simulink model "OffboardAPI"  (R2021b)
settings: Solver=ode4  StartTime=0.0  StopTime=inf  FixedStep=0.01  RelTol=1e-3
PreLoadFcn:
  | filepath  = fileparts(get_param(bdroot, 'FileName'))
  | cd(filepath);
undefined symbols (not defined in the file): Busy, Earth, Wait, WGS84
libraries: etargetslib x10, slrealtimeiplib x2, dspnetwork x2, slrealtimeutilitieslib x1, aerolibanimutils x1, aerolibtransform2 x1
settings Model: Creator=dream  LastModifiedBy=Lenovo
settings SolverCC: AlgebraicLoopSolver=TrustRegion
settings DataIOCC: ReturnWorkspaceOutputs=off
settings DebuggingCC: SFMachineParentedDataDiag=warning  ArithmeticOperatorsInVariantConditions=warning
settings SFSimCC: SimUseLocalCustomCode=off  CustomCodeUndefinedFunction=UseInterfaceOnly
settings RTWCC: RTWUseLocalCustomCode=off

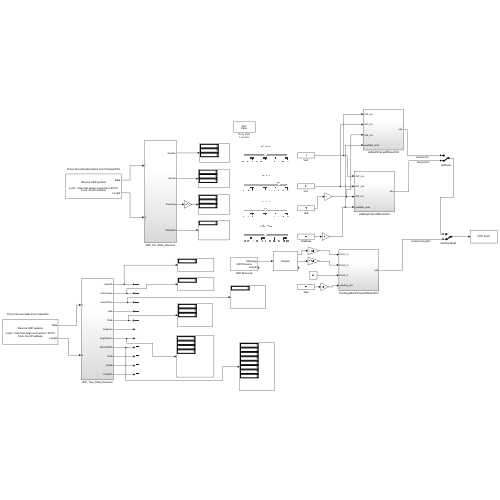
[thumbnail: Simulink's stored preview of the top-level diagram]
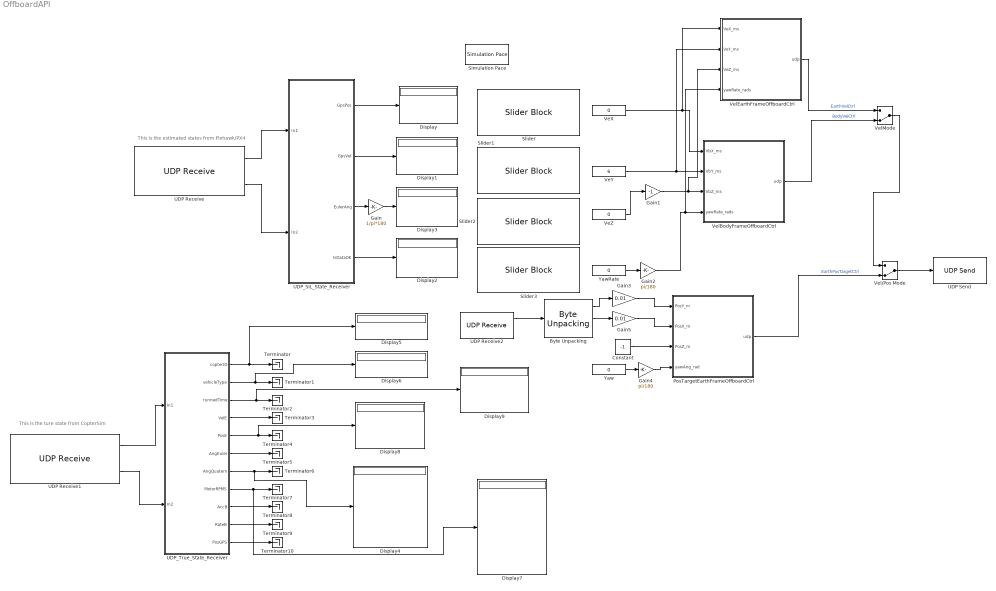
== system OffboardAPI ==
  note: This is the estimated states from Pixhawk/PX4
  note: This is the ture state from CopterSim
  Byte Unpacking : slrealtimeutilitieslib/Byte Unpacking  MaskUnpackedDataTypes={'double','double','double'}  MaskUnpackedDataSizes={[1],[1],[1]}  MaskAlignment=1
      settings: SourceProductBaseCode=XP
  Constant : Constant  Value=-1
  Display{,1..9} (10 alike) : Display
  Gain : Gain  Gain=1/pi*180
  Gain1 : Gain  Gain=-1
  Gain2 : Gain  Gain=pi/180
  Gain3 : Gain  Gain=0.01
  Gain4 : Gain  Gain=pi/180
  Gain5 : Gain  Gain=0.01
  PosTargetEarthFrameOffboardCtrl : Subsystem
  Simulation Pace : aerolibanimutils/Simulation Pace  SimulationPace=1  SleepMode=Busy-Wait  OutputPaceError=off  SampleTime=-1
  Slider : SliderBlock  ScaleMin=-10  ScaleMax=10
  Slider1 : SliderBlock  ScaleMin=-10  ScaleMax=10
  Slider2 : SliderBlock  ScaleMin=-10  ScaleMax=10
  Slider3 : SliderBlock  ScaleMin=-180  ScaleMax=180
  Terminator{,1..10} (11 alike) : Terminator
  UDP Receive : slrealtimeiplib/UDP Receive  useHostTargetConn=on  ipAddress=10.10.10.15  localPort=20101  rcvWidth=125  rcvFmAny=on  fmAddress=0.0.0.0  sampleTime=-1
      settings: SourceProductBaseCode=XP
  UDP Receive1 : slrealtimeiplib/UDP Receive  useHostTargetConn=on  ipAddress=10.10.10.15  localPort=30101  rcvWidth=250  rcvFmAny=on  fmAddress=0.0.0.0  sampleTime=-1
      settings: SourceProductBaseCode=XP
  UDP Receive2 : dspnetwork/UDP Receive  localURL='0.0.0.0'  localPort=1230  remoteURL='127.0.0.1'  remotePort=-1  recvBufferSize=24  dims=3  signalDatatype=double  isComplex=off  isVarSize=off  showBlockingTime=off  blockingTime=0  sampletime=-1  blockPlatform=[]
  UDP Send : dspnetwork/UDP Send  remoteURL='127.0.0.1'  remotePort=20100  localURL='0.0.0.0'  localPortSource=Automatically determine  localPort=-1  sendBufferSize=8192  sampletime=-1  blockPlatform=[]  separateLengthPort=0
  UDP_SIL_State_Receiver : Subsystem
  UDP_True_State_Receiver : Subsystem
  VeX : Constant  Value=0
  VeY : Constant  Value=6
  VeZ : Constant  Value=0
  Vel/Pos Mode : ManualSwitch  CurrentSetting=0
  VelBodyFrameOffboardCtrl : Subsystem
  VelEarthFrameOffboardCtrl : Subsystem
  VelMode : ManualSwitch  CurrentSetting=0
  Yaw : Constant  Value=0
  YawRate : Constant  Value=0
  wires:
  UDP Receive/1 -> UDP_SIL_State_Receiver/1(In1)
  UDP Receive/2 -> UDP_SIL_State_Receiver/2(In2)
  UDP_SIL_State_Receiver/1(GpsPos) -> Display/1
  UDP_SIL_State_Receiver/2(GpsVel) -> Display1/1
  UDP_SIL_State_Receiver/3(EulerAng) -> Gain/1
  VeX/1 -> VelEarthFrameOffboardCtrl/1(VeX_ms), VelBodyFrameOffboardCtrl/1(VbX_ms)
  VeY/1 -> VelEarthFrameOffboardCtrl/2(VeY_ms), VelBodyFrameOffboardCtrl/2(VbY_ms)
  VeZ/1 -> Gain1/1
  YawRate/1 -> Gain2/1
  VelBodyFrameOffboardCtrl/1(udp) -> VelMode/2  "BodyVelCtrl"
  Gain/1 -> Display3/1
  Gain1/1 -> VelEarthFrameOffboardCtrl/3(VeZ_ms), VelBodyFrameOffboardCtrl/3(VbZ_ms)
  UDP_SIL_State_Receiver/4(IsDataOK) -> Display2/1
  Gain2/1 -> VelEarthFrameOffboardCtrl/4(yawRate_rads), VelBodyFrameOffboardCtrl/4(yawRate_rads)
  Yaw/1 -> Gain4/1
  PosTargetEarthFrameOffboardCtrl/1(udp) -> Vel/Pos Mode/2  "EarthPosTargetCtrl"
  Vel/Pos Mode/1 -> UDP Send/1
  Gain4/1 -> PosTargetEarthFrameOffboardCtrl/4(yawAng_rad)
  VelEarthFrameOffboardCtrl/1(udp) -> VelMode/1  "EarthVelCtrl"
  VelMode/1 -> Vel/Pos Mode/1
  UDP_True_State_Receiver/2(vehicleType) -> Display6/1, Terminator1/1
  UDP Receive1/2 -> UDP_True_State_Receiver/2(In2)
  UDP_True_State_Receiver/11(PosGPS) -> Terminator10/1
  UDP_True_State_Receiver/10(RateB) -> Terminator9/1
  UDP_True_State_Receiver/8(MotorRPMS) -> Display7/1, Terminator7/1
  UDP_True_State_Receiver/9(AccB) -> Terminator8/1
  UDP_True_State_Receiver/1(copterID) -> Display5/1, Terminator/1
  UDP_True_State_Receiver/7(AngQuatern) -> Display4/1, Terminator6/1
  UDP_True_State_Receiver/3(runnedTime) -> Display9/1, Terminator2/1
  UDP_True_State_Receiver/5(PosE) -> Display8/1, Terminator4/1
  UDP_True_State_Receiver/6(AngEuler) -> Terminator5/1
  UDP_True_State_Receiver/4(VelE) -> Terminator3/1
  UDP Receive1/1 -> UDP_True_State_Receiver/1(In1)
  Byte Unpacking/1 -> Gain3/1
  Byte Unpacking/2 -> Gain5/1
  UDP Receive2/1 -> Byte Unpacking/1
  Gain3/1 -> PosTargetEarthFrameOffboardCtrl/1(PosY_m)
  Gain5/1 -> PosTargetEarthFrameOffboardCtrl/2(PosX_m)
  Constant/1 -> PosTargetEarthFrameOffboardCtrl/3(PosZ_m)

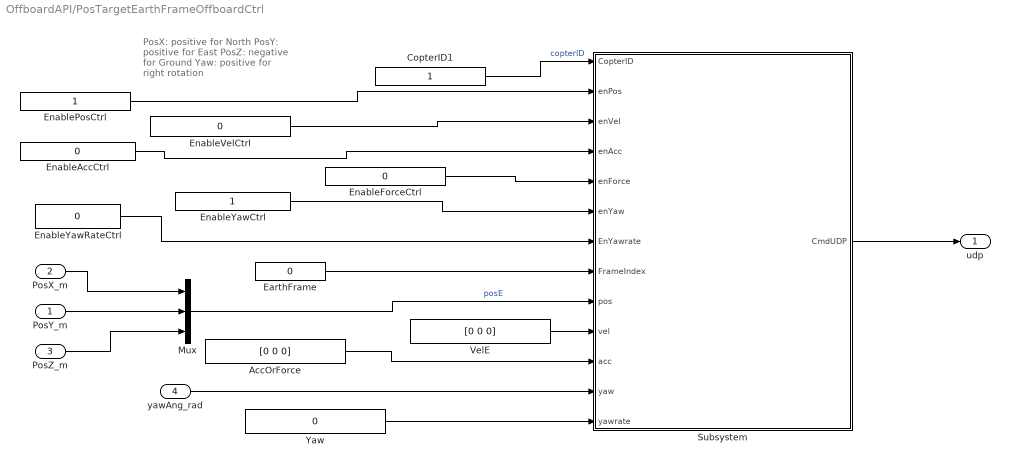
== system OffboardAPI/PosTargetEarthFrameOffboardCtrl ==
  note: PosX: positive for North
      | PosY: positive for East
      | PosZ: negative for Ground
      | Yaw: positive for right rotation
  PosY_m : Inport
  PosX_m : Inport  Port=2
  PosZ_m : Inport  Port=3
  yawAng_rad : Inport  Port=4  PortDimensions=1
  AccOrForce : Constant  Value=[0 0 0]
  CopterID1 : Constant
  EarthFrame : Constant  Value=0
  EnableAccCtrl : Constant  Value=0
  EnableForceCtrl : Constant  Value=0
  EnablePosCtrl : Constant
  EnableVelCtrl : Constant  Value=0
  EnableYawCtrl : Constant
  EnableYawRateCtrl : Constant  Value=0
  Mux : Mux  Inputs=3
  Subsystem : Subsystem
  VelE : Constant  Value=[0 0 0]
  Yaw : Constant  Value=0
  udp : Outport  VectorParamsAs1DForOutWhenUnconnected=off
  wires:
  Subsystem/1(CmdUDP) -> udp/1
  Yaw/1 -> Subsystem/13(yawrate)
  EnableYawRateCtrl/1 -> Subsystem/7(EnYawrate)
  EnableYawCtrl/1 -> Subsystem/6(enYaw)
  EnableAccCtrl/1 -> Subsystem/4(enAcc)
  Mux/1 -> Subsystem/9(pos)  "posE"
  EarthFrame/1 -> Subsystem/8(FrameIndex)
  yawAng_rad/1 -> Subsystem/12(yaw)
  AccOrForce/1 -> Subsystem/11(acc)
  EnableVelCtrl/1 -> Subsystem/3(enVel)
  EnableForceCtrl/1 -> Subsystem/5(enForce)
  CopterID1/1 -> Subsystem/1(CopterID)  "copterID"
  EnablePosCtrl/1 -> Subsystem/2(enPos)
  VelE/1 -> Subsystem/10(vel)
  PosY_m/1 -> Mux/2
  PosX_m/1 -> Mux/1
  PosZ_m/1 -> Mux/3

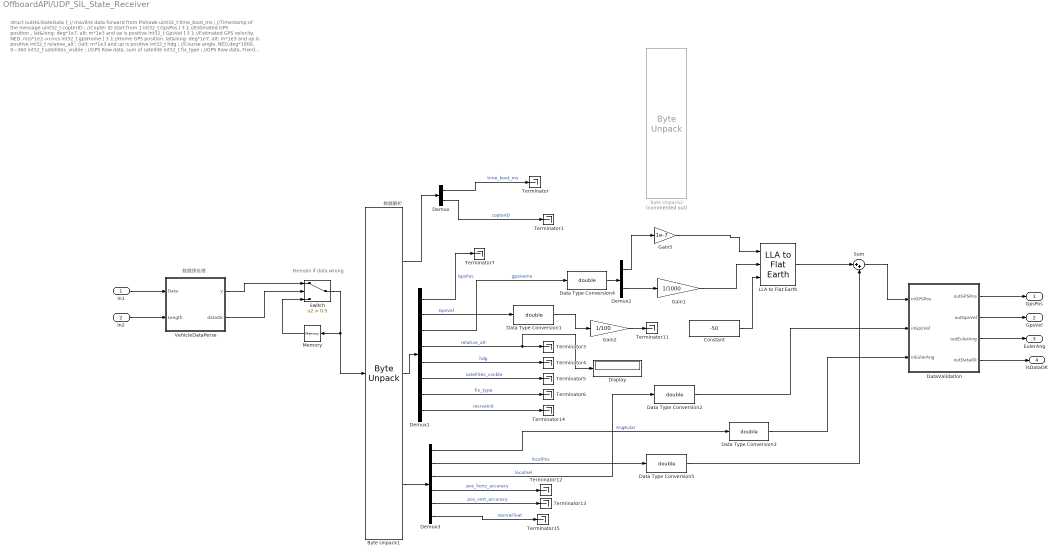
== system OffboardAPI/UDP_SIL_State_Receiver ==
  note: 数据解析
  note: 数据预处理
  note: Remain if data wrong
  note: struct outHILStateData { // mavlink data forward from Pixhawk
      | uint32_t time_boot_ms ; //Timestamp of the message
      | uint32_t copterID ; //Copter ID start from 1
      | int32_t GpsPos [ 3 ]; //Estimated GPS position，lat&long: deg*1e7, alt: m*1e3 and up is positive
      | int32_t GpsVel [ 3 ]; //Estimated GPS velocity, NED, m/s*1e2->cm/s
      | int32_t gpsHome [ 3 ]; //Home GPS position, lat&long: deg*1e7, alt: m*1e3 and up is positive
      | int32_t relative_alt ; //alt: m*1e3 and up is positive
      | int32_t hdg ; //Course angle, NED,deg*1000, 0~360
      | int32_t satellites_visible ; //GPS Raw data, sum of satellite
      | int32_t fix_type ; //GPS Raw data, Fixed type, 3 for fixed (good precision)
      | int32_t resrveInit ; //Int, reserve for the future use
      | float AngEular [ 3 ]; //Estimated Euler angle, unit: rad/s
      | float localPos [ 3 ]; //Estimated locoal position, NED, unit: m
      | float localVel [ 3 ]; //Estimated locoal velocity, NED, unit: m/s
      | float pos_horiz_accuracy ; //GPS horizontal accuracy, unit: m
      | float pos_vert_accuracy ; //GPS vertical accuracy, unit: m
      | float resrveFloat ; //float,reserve for the future use
      | }
  In1 : Inport
  In2 : Inport  Port=2
  Byte Unpack1 : etargetslib/Byte Unpack  dimensions={2,14,12}  datatypes={'uint32','int32','single'}  byteAlign=8
  Byte Unpack2 : etargetslib/Byte Unpack  Commented=on  dimensions={1,1,1,3,3,3,4,8,3,3,3}  datatypes={'int32','int32','double','single','single','single','single','single','single','single','double'}  byteAlign=1
  Constant : Constant  Value=-50
  Data Type Conversion{1..5} (5 alike) : DataTypeConversion  OutDataTypeStr=double
  DataValidation : MATLAB Function  TreatAsAtomicUnit=on
  Demux : Demux  Outputs=2
  Demux1 : Demux  Outputs=[3,3,3,1,1,1,1,1]
  Demux2 : Demux  Outputs=[2,1]
  Demux3 : Demux  Outputs=[3,3,3,1,1,1]
  Display : Display
  Gain1 : Gain  Gain=1/1000
  Gain2 : Gain  Gain=1/100
  Gain5 : Gain  Gain=1e-7
  LLA to Flat Earth : aerolibtransform2/LLA to Flat Earth  units=Metric (MKS)  ptype=Earth (WGS84)  F=1/298.257223563  R=6378137  refPosPort=off  LL0=[40.1540302 116.259368300000]  psi=0
      settings: SourceProductBaseCode=AE
  Memory : Memory  InitialCondition=uint8(zeros(112,1))
  Sum : Sum  Inputs=|++
  Switch : Switch  Criteria=u2 > Threshold  Threshold=0.5
  Terminator{,1,3..7,11..15} (12 alike) : Terminator
  VehicleDataPerse : MATLAB Function  TreatAsAtomicUnit=on
  GpsPos : Outport  VectorParamsAs1DForOutWhenUnconnected=off
  GpsVel : Outport  Port=2  VectorParamsAs1DForOutWhenUnconnected=off
  EulerAng : Outport  Port=3  VectorParamsAs1DForOutWhenUnconnected=off
  IsDataOK : Outport  Port=4  VectorParamsAs1DForOutWhenUnconnected=off
  wires:
  VehicleDataPerse/2(dataOk) -> Switch/2
  In2/1 -> VehicleDataPerse/2(Length)
  In1/1 -> VehicleDataPerse/1(Data)
  VehicleDataPerse/1(y) -> Switch/1
  Switch/1 -> Memory/1, Byte Unpack1/1
  Memory/1 -> Switch/3
  Byte Unpack1/1 -> Demux/1
  Demux/1 -> Terminator/1  "time_boot_ms"
  Demux/2 -> Terminator1/1  "copterID"
  Byte Unpack1/2 -> Demux1/1
  Demux1/2 -> Data Type Conversion1/1  "GpsVel"
  Demux2/1 -> Gain5/1
  Demux2/2 -> Gain1/1
  Gain1/1 -> LLA to Flat Earth/2
  Demux1/1 -> Terminator7/1  "GpsPos"
  LLA to Flat Earth/1 -> Sum/1
  Data Type Conversion1/1 -> Gain2/1
  Data Type Conversion3/1 -> DataValidation/3(inEulerAng)
  Gain5/1 -> LLA to Flat Earth/1
  Data Type Conversion4/1 -> Demux2/1
  Byte Unpack1/3 -> Demux3/1
  Demux1/3 -> Data Type Conversion4/1  "gpsHome"
  Demux1/4 -> Display/1, Terminator3/1  "relative_alt"
  Demux1/5 -> Terminator4/1  "hdg"
  Demux1/6 -> Terminator5/1  "satellites_visible"
  Demux1/7 -> Terminator6/1  "fix_type"
  Demux3/1 -> Data Type Conversion3/1  "AngEular"
  Demux3/2 -> Data Type Conversion5/1  "localPos"
  Demux3/3 -> Data Type Conversion2/1  "localVel"
  Demux3/4 -> Terminator12/1  "pos_horiz_accuracy"
  Demux3/5 -> Terminator13/1  "pos_vert_accuracy"
  Demux1/8 -> Terminator14/1  "resrveInit"
  Demux3/6 -> Terminator15/1  "resrveFloat"
  Constant/1 -> LLA to Flat Earth/3
  DataValidation/1(outGPSPos) -> GpsPos/1
  DataValidation/2(outGpsVel) -> GpsVel/1
  DataValidation/3(outEulerAng) -> EulerAng/1
  DataValidation/4(outDataOk) -> IsDataOK/1
  Data Type Conversion2/1 -> DataValidation/2(inGpsVel)
  Gain2/1 -> Terminator11/1
  Data Type Conversion5/1 -> Sum/2
  Sum/1 -> DataValidation/1(inGPSPos)

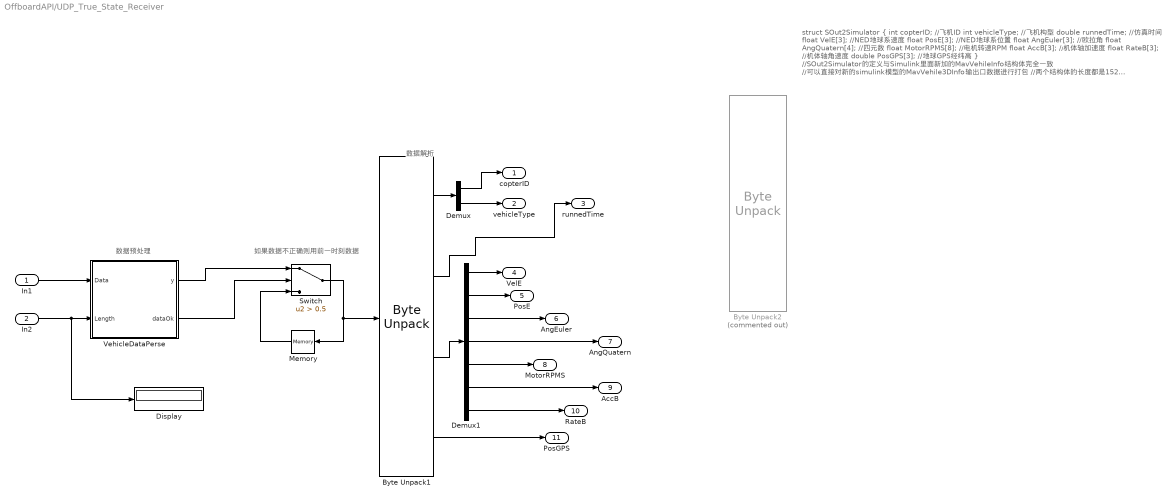
== system OffboardAPI/UDP_True_State_Receiver ==
  note: 数据解析
  note: 数据预处理
  note: 如果数据不正确则用前一时刻数据
  note: struct SOut2Simulator
      | {
      | int copterID; //飞机ID
      | int vehicleType; //飞机构型
      | double runnedTime; //仿真时间
      | float VelE[3]; //NED地球系速度
      | float PosE[3]; //NED地球系位置
      | float AngEuler[3]; //欧拉角
      | float AngQuatern[4]; //四元数
      | float MotorRPMS[8]; //电机转速RPM
      | float AccB[3]; //机体轴加速度
      | float RateB[3]; //机体轴角速度
      | double PosGPS[3]; //地球GPS经纬高
      | }
      |
      | //SOut2Simulator的定义与Simulink里面新加的MavVehileInfo结构体完全一致
      | //可以直接对新的simulink模型的MavVehile3DInfo输出口数据进行打包
      | //两个结构体的长度都是152
      | sizeof(SOut2Simulator) = sizeof(MavVehileInfo) = 152
      |
      | 打包封装的结构体为
      | typedef struct _netDataShort
      | {
      | TargetType tg; //这里目前随便填，写1即可 uint32
      | int len; //这个长度为传输结构体长度，目前是152
      | char payload[192]; //这里面前152位存放了SOut2Simulator结构体数据，后面的40位保留
      | }netDataShort;
      |
      | //UDP包的总长度为200
      | sizeof(netDataShort) = 200
      |
      | //发送的UDP端口号为：20010
  In1 : Inport
  In2 : Inport  Port=2
  Byte Unpack1 : etargetslib/Byte Unpack  dimensions={2,1,27,3}  datatypes={'int32','double','single','double'}  byteAlign=8
  Byte Unpack2 : etargetslib/Byte Unpack  Commented=on  dimensions={1,1,1,3,3,3,4,8,3,3,3}  datatypes={'int32','int32','double','single','single','single','single','single','single','single','double'}  byteAlign=1
  Demux : Demux  Outputs=2
  Demux1 : Demux  Outputs=[3,3,3,4,8,3,3]
  Display : Display
  Memory : Memory  InitialCondition=uint8(zeros(152,1))
  Switch : Switch  Criteria=u2 > Threshold  Threshold=0.5
  VehicleDataPerse : MATLAB Function  TreatAsAtomicUnit=on
  copterID : Outport  VectorParamsAs1DForOutWhenUnconnected=off
  vehicleType : Outport  Port=2  VectorParamsAs1DForOutWhenUnconnected=off
  runnedTime : Outport  Port=3  VectorParamsAs1DForOutWhenUnconnected=off
  VelE : Outport  Port=4  VectorParamsAs1DForOutWhenUnconnected=off
  PosE : Outport  Port=5  VectorParamsAs1DForOutWhenUnconnected=off
  AngEuler : Outport  Port=6  VectorParamsAs1DForOutWhenUnconnected=off
  AngQuatern : Outport  Port=7  VectorParamsAs1DForOutWhenUnconnected=off
  MotorRPMS : Outport  Port=8  VectorParamsAs1DForOutWhenUnconnected=off
  AccB : Outport  Port=9  VectorParamsAs1DForOutWhenUnconnected=off
  RateB : Outport  Port=10  VectorParamsAs1DForOutWhenUnconnected=off
  PosGPS : Outport  Port=11  VectorParamsAs1DForOutWhenUnconnected=off
  wires:
  VehicleDataPerse/2(dataOk) -> Switch/2
  In2/1 -> Display/1, VehicleDataPerse/2(Length)
  In1/1 -> VehicleDataPerse/1(Data)
  VehicleDataPerse/1(y) -> Switch/1
  Switch/1 -> Memory/1, Byte Unpack1/1
  Memory/1 -> Switch/3
  Byte Unpack1/1 -> Demux/1
  Demux/1 -> copterID/1
  Demux/2 -> vehicleType/1
  Byte Unpack1/2 -> runnedTime/1
  Byte Unpack1/3 -> Demux1/1
  Demux1/1 -> VelE/1
  Demux1/2 -> PosE/1
  Demux1/3 -> AngEuler/1
  Demux1/4 -> AngQuatern/1
  Demux1/5 -> MotorRPMS/1
  Demux1/6 -> AccB/1
  Demux1/7 -> RateB/1
  Byte Unpack1/4 -> PosGPS/1

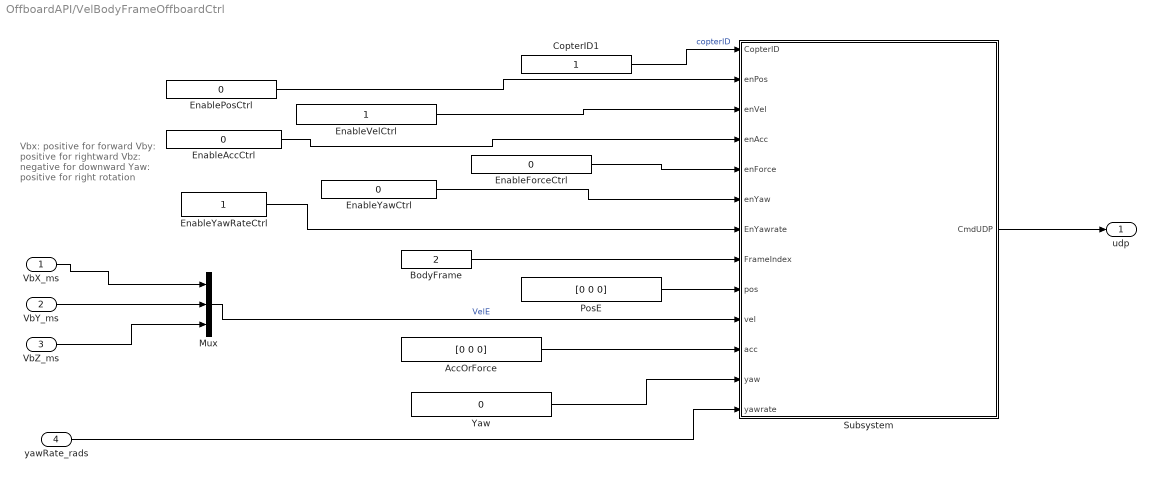
== system OffboardAPI/VelBodyFrameOffboardCtrl ==
  note: Vbx: positive for forward
      | Vby: positive for rightward
      | Vbz: negative for downward
      | Yaw: positive for right rotation
  VbX_ms : Inport
  VbY_ms : Inport  Port=2
  VbZ_ms : Inport  Port=3
  yawRate_rads : Inport  Port=4  PortDimensions=1
  AccOrForce : Constant  Value=[0 0 0]
  BodyFrame : Constant  Value=2
  CopterID1 : Constant
  EnableAccCtrl : Constant  Value=0
  EnableForceCtrl : Constant  Value=0
  EnablePosCtrl : Constant  Value=0
  EnableVelCtrl : Constant
  EnableYawCtrl : Constant  Value=0
  EnableYawRateCtrl : Constant
  Mux : Mux  Inputs=3
  PosE : Constant  Value=[0 0 0]
  Subsystem : Subsystem
  Yaw : Constant  Value=0
  udp : Outport  VectorParamsAs1DForOutWhenUnconnected=off
  wires:
  Subsystem/1(CmdUDP) -> udp/1
  Yaw/1 -> Subsystem/12(yaw)
  EnableYawRateCtrl/1 -> Subsystem/7(EnYawrate)
  EnableYawCtrl/1 -> Subsystem/6(enYaw)
  EnableAccCtrl/1 -> Subsystem/4(enAcc)
  Mux/1 -> Subsystem/10(vel)  "VelE"
  BodyFrame/1 -> Subsystem/8(FrameIndex)
  yawRate_rads/1 -> Subsystem/13(yawrate)
  AccOrForce/1 -> Subsystem/11(acc)
  EnableVelCtrl/1 -> Subsystem/3(enVel)
  EnableForceCtrl/1 -> Subsystem/5(enForce)
  CopterID1/1 -> Subsystem/1(CopterID)  "copterID"
  EnablePosCtrl/1 -> Subsystem/2(enPos)
  PosE/1 -> Subsystem/9(pos)
  VbY_ms/1 -> Mux/2
  VbX_ms/1 -> Mux/1
  VbZ_ms/1 -> Mux/3

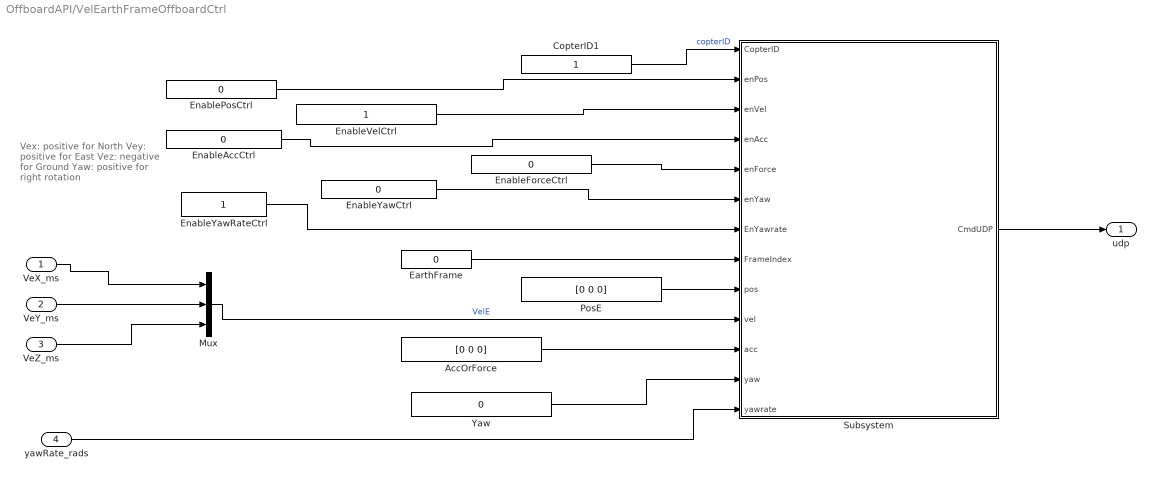
== system OffboardAPI/VelEarthFrameOffboardCtrl ==
  note: Vex: positive for North
      | Vey: positive for East
      | Vez: negative for Ground
      | Yaw: positive for right rotation
  VeX_ms : Inport
  VeY_ms : Inport  Port=2
  VeZ_ms : Inport  Port=3
  yawRate_rads : Inport  Port=4  PortDimensions=1
  AccOrForce : Constant  Value=[0 0 0]
  CopterID1 : Constant
  EarthFrame : Constant  Value=0
  EnableAccCtrl : Constant  Value=0
  EnableForceCtrl : Constant  Value=0
  EnablePosCtrl : Constant  Value=0
  EnableVelCtrl : Constant
  EnableYawCtrl : Constant  Value=0
  EnableYawRateCtrl : Constant
  Mux : Mux  Inputs=3
  PosE : Constant  Value=[0 0 0]
  Subsystem : Subsystem
  Yaw : Constant  Value=0
  udp : Outport  VectorParamsAs1DForOutWhenUnconnected=off
  wires:
  Subsystem/1(CmdUDP) -> udp/1
  Yaw/1 -> Subsystem/12(yaw)
  EnableYawRateCtrl/1 -> Subsystem/7(EnYawrate)
  EnableYawCtrl/1 -> Subsystem/6(enYaw)
  EnableAccCtrl/1 -> Subsystem/4(enAcc)
  Mux/1 -> Subsystem/10(vel)  "VelE"
  EarthFrame/1 -> Subsystem/8(FrameIndex)
  yawRate_rads/1 -> Subsystem/13(yawrate)
  AccOrForce/1 -> Subsystem/11(acc)
  EnableVelCtrl/1 -> Subsystem/3(enVel)
  EnableForceCtrl/1 -> Subsystem/5(enForce)
  CopterID1/1 -> Subsystem/1(CopterID)  "copterID"
  EnablePosCtrl/1 -> Subsystem/2(enPos)
  PosE/1 -> Subsystem/9(pos)
  VeY_ms/1 -> Mux/2
  VeX_ms/1 -> Mux/1
  VeZ_ms/1 -> Mux/3

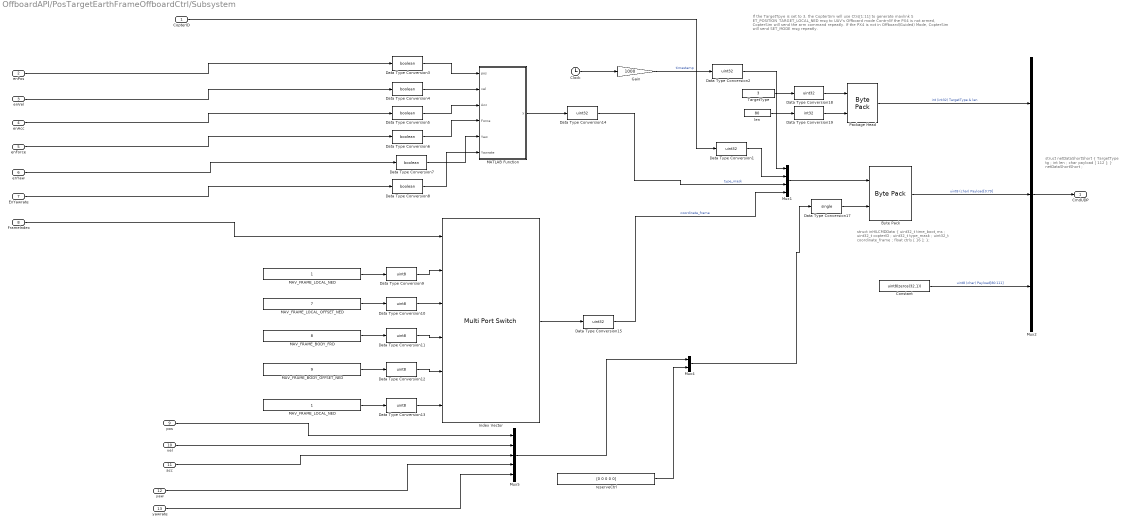
== system OffboardAPI/PosTargetEarthFrameOffboardCtrl/Subsystem ==
  note: struct netDataShortShort {
      | TargetType tg ;
      | int len ;
      | char payload [ 112 ];
      | } netDataShortShort ;
  note: struct inHILCMDData {
      | uint32_t time_boot_ms ;
      | uint32_t copterID ;
      | uint32_t type_mask ;
      | uint32_t coordinate_frame ;
      | float ctrls [ 16 ];
      | };
  note: If the TargetTpye is set to 3, the CopterSim will use Ctrs[1:11] to generate mavlink S ET_POSITION_TARGET_LOCAL_NED msg to UAV's Offboard mode Control，
      | If the PX4 is not armed, CopterSim will send the arm command repeatly. If the PX4 is not in Offboard(Guided) Mode, CopterSim will send SET_MODE msg repeatly.
  CopterID : Inport
  enPos : Inport  Port=2
  enVel : Inport  Port=3
  enAcc : Inport  Port=4
  enForce : Inport  Port=5
  enYaw : Inport  Port=6
  EnYawrate : Inport  Port=7
  FrameIndex : Inport  Port=8
  pos : Inport  Port=9  PortDimensions=3
  vel : Inport  Port=10  PortDimensions=3
  acc : Inport  Port=11  PortDimensions=3
  yaw : Inport  Port=12  PortDimensions=1
  yawrate : Inport  Port=13  PortDimensions=1
  Byte Pack : etargetslib/Byte Pack  datatypes={'uint32','single'}  byteAlign=1
  Clock : Clock
  Constant : Constant  Value=uint8(zeros(32,1))
  Data Type Conversion{1,14..15,18} (4 alike) : DataTypeConversion  OutDataTypeStr=uint32
  Data Type Conversion{9..13} (5 alike) : DataTypeConversion  OutDataTypeStr=uint8
  Data Type Conversion17 : DataTypeConversion  OutDataTypeStr=single  LockScale=on
  Data Type Conversion19 : DataTypeConversion  OutDataTypeStr=int32
  Data Type Conversion2 : DataTypeConversion  OutDataTypeStr=uint32  RndMeth=Round
  Data Type Conversion{3..8} (6 alike) : DataTypeConversion  OutDataTypeStr=boolean
  Gain : Gain  Gain=1000
  Index Vector : MultiPortSwitch  DataPortOrder=Zero-based contiguous  Inputs=5  zeroidx=on
  MATLAB Function : MATLAB Function  TreatAsAtomicUnit=on
  MAV_FRAME_BODY_FRD : Constant  Value=8
  "MAV_FRAME_BODY_OFFSET_NED " : Constant  Value=9
  MAV_FRAME_LOCAL_NED : Constant
  "MAV_FRAME_LOCAL_NED " : Constant
  MAV_FRAME_LOCAL_OFFSET_NED : Constant  Value=7
  Mux1 : Mux
  Mux2 : Mux  Inputs=3
  Mux4 : Mux  Inputs=2
  Mux5 : Mux  Inputs=5
  Package Head : etargetslib/Byte Pack  datatypes={'uint32','int32'}  byteAlign=4
  TargetType : Constant  Value=3  OutDataTypeStr=Inherit: Inherit via back propagation
  len : Constant  Value=80  OutDataTypeStr=Inherit: Inherit via back propagation
  reserveCtrl : Constant  Value=[0 0 0 0 0]
  CmdUDP : Outport  VectorParamsAs1DForOutWhenUnconnected=off
  wires:
  Data Type Conversion7/1 -> MATLAB Function/5(Yaw)
  Data Type Conversion6/1 -> MATLAB Function/4(Force)
  MATLAB Function/1(y) -> Data Type Conversion14/1
  vel/1 -> Mux5/2
  MAV_FRAME_BODY_FRD/1 -> Data Type Conversion11/1
  Data Type Conversion3/1 -> MATLAB Function/1(pos)
  Data Type Conversion5/1 -> MATLAB Function/3(Acc)
  Data Type Conversion4/1 -> MATLAB Function/2(vel)
  Data Type Conversion8/1 -> MATLAB Function/6(Yawrate)
  enAcc/1 -> Data Type Conversion5/1
  enYaw/1 -> Data Type Conversion7/1
  EnYawrate/1 -> Data Type Conversion8/1
  enForce/1 -> Data Type Conversion6/1
  "MAV_FRAME_LOCAL_NED "/1 -> Data Type Conversion9/1
  enPos/1 -> Data Type Conversion3/1
  Data Type Conversion9/1 -> Index Vector/2
  Mux5/1 -> Mux4/1
  Data Type Conversion10/1 -> Index Vector/3
  Data Type Conversion15/1 -> Mux1/4  "coordinate_frame"
  Constant/1 -> Mux2/3  "uint8 (char) Payload[80:111]"
  Data Type Conversion18/1 -> Package Head/1
  Clock/1 -> Gain/1
  len/1 -> Data Type Conversion19/1
  Data Type Conversion17/1 -> Byte Pack/2
  Data Type Conversion14/1 -> Mux1/3  "type_mask"
  Mux1/1 -> Byte Pack/1
  Package Head/1 -> Mux2/1  "int (int32) TargetType & len"
  Mux4/1 -> Data Type Conversion17/1
  TargetType/1 -> Data Type Conversion18/1
  Mux2/1 -> CmdUDP/1
  CopterID/1 -> Data Type Conversion1/1
  Gain/1 -> Data Type Conversion2/1  "timestamp"
  Data Type Conversion19/1 -> Package Head/2
  pos/1 -> Mux5/1
  Byte Pack/1 -> Mux2/2  "uint8 (char) Payload[0:79]"
  Data Type Conversion13/1 -> Index Vector/6
  Data Type Conversion12/1 -> Index Vector/5
  reserveCtrl/1 -> Mux4/2
  acc/1 -> Mux5/3
  FrameIndex/1 -> Index Vector/1
  Index Vector/1 -> Data Type Conversion15/1
  MAV_FRAME_LOCAL_NED/1 -> Data Type Conversion13/1
  MAV_FRAME_LOCAL_OFFSET_NED/1 -> Data Type Conversion10/1
  Data Type Conversion11/1 -> Index Vector/4
  "MAV_FRAME_BODY_OFFSET_NED "/1 -> Data Type Conversion12/1
  enVel/1 -> Data Type Conversion4/1
  yaw/1 -> Mux5/4
  yawrate/1 -> Mux5/5
  Data Type Conversion1/1 -> Mux1/2
  Data Type Conversion2/1 -> Mux1/1

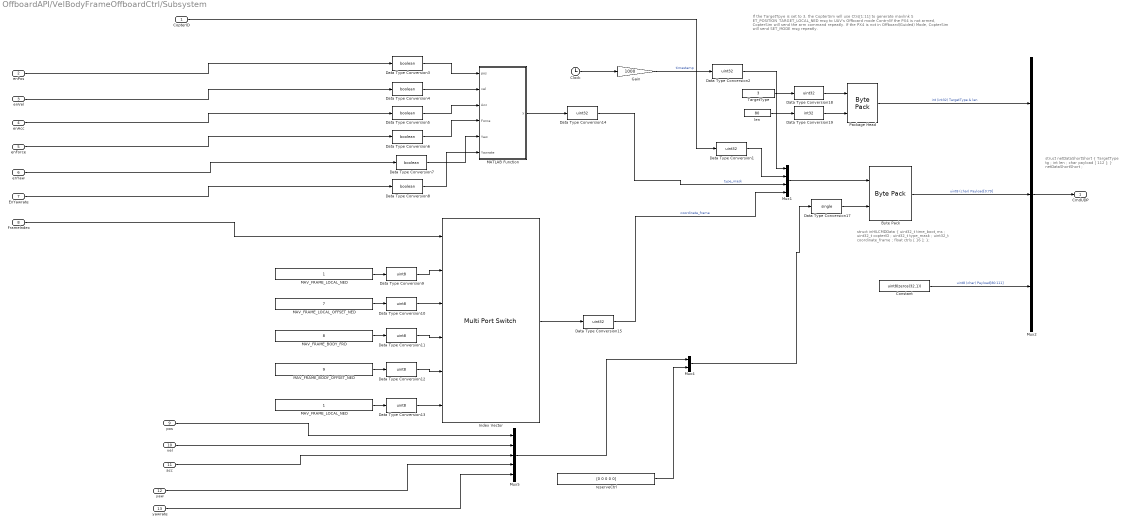
== system OffboardAPI/VelBodyFrameOffboardCtrl/Subsystem ==
  note: struct netDataShortShort {
      | TargetType tg ;
      | int len ;
      | char payload [ 112 ];
      | } netDataShortShort ;
  note: struct inHILCMDData {
      | uint32_t time_boot_ms ;
      | uint32_t copterID ;
      | uint32_t type_mask ;
      | uint32_t coordinate_frame ;
      | float ctrls [ 16 ];
      | };
  note: If the TargetTpye is set to 3, the CopterSim will use Ctrs[1:11] to generate mavlink S ET_POSITION_TARGET_LOCAL_NED msg to UAV's Offboard mode Control，
      | If the PX4 is not armed, CopterSim will send the arm command repeatly. If the PX4 is not in Offboard(Guided) Mode, CopterSim will send SET_MODE msg repeatly.
  CopterID : Inport
  enPos : Inport  Port=2
  enVel : Inport  Port=3
  enAcc : Inport  Port=4
  enForce : Inport  Port=5
  enYaw : Inport  Port=6
  EnYawrate : Inport  Port=7
  FrameIndex : Inport  Port=8
  pos : Inport  Port=9  PortDimensions=3
  vel : Inport  Port=10  PortDimensions=3
  acc : Inport  Port=11  PortDimensions=3
  yaw : Inport  Port=12  PortDimensions=1
  yawrate : Inport  Port=13  PortDimensions=1
  Byte Pack : etargetslib/Byte Pack  datatypes={'uint32','single'}  byteAlign=1
  Clock : Clock
  Constant : Constant  Value=uint8(zeros(32,1))
  Data Type Conversion{1,14..15,18} (4 alike) : DataTypeConversion  OutDataTypeStr=uint32
  Data Type Conversion{9..13} (5 alike) : DataTypeConversion  OutDataTypeStr=uint8
  Data Type Conversion17 : DataTypeConversion  OutDataTypeStr=single  LockScale=on
  Data Type Conversion19 : DataTypeConversion  OutDataTypeStr=int32
  Data Type Conversion2 : DataTypeConversion  OutDataTypeStr=uint32  RndMeth=Round
  Data Type Conversion{3..8} (6 alike) : DataTypeConversion  OutDataTypeStr=boolean
  Gain : Gain  Gain=1000
  Index Vector : MultiPortSwitch  DataPortOrder=Zero-based contiguous  Inputs=5  zeroidx=on
  MATLAB Function : MATLAB Function  TreatAsAtomicUnit=on
  MAV_FRAME_BODY_FRD : Constant  Value=8
  "MAV_FRAME_BODY_OFFSET_NED " : Constant  Value=9
  MAV_FRAME_LOCAL_NED : Constant
  "MAV_FRAME_LOCAL_NED " : Constant
  MAV_FRAME_LOCAL_OFFSET_NED : Constant  Value=7
  Mux1 : Mux
  Mux2 : Mux  Inputs=3
  Mux4 : Mux  Inputs=2
  Mux5 : Mux  Inputs=5
  Package Head : etargetslib/Byte Pack  datatypes={'uint32','int32'}  byteAlign=4
  TargetType : Constant  Value=3  OutDataTypeStr=Inherit: Inherit via back propagation
  len : Constant  Value=80  OutDataTypeStr=Inherit: Inherit via back propagation
  reserveCtrl : Constant  Value=[0 0 0 0 0]
  CmdUDP : Outport  VectorParamsAs1DForOutWhenUnconnected=off
  wires:
  Data Type Conversion7/1 -> MATLAB Function/5(Yaw)
  Data Type Conversion6/1 -> MATLAB Function/4(Force)
  MATLAB Function/1(y) -> Data Type Conversion14/1
  vel/1 -> Mux5/2
  MAV_FRAME_BODY_FRD/1 -> Data Type Conversion11/1
  Data Type Conversion3/1 -> MATLAB Function/1(pos)
  Data Type Conversion5/1 -> MATLAB Function/3(Acc)
  Data Type Conversion4/1 -> MATLAB Function/2(vel)
  Data Type Conversion8/1 -> MATLAB Function/6(Yawrate)
  enAcc/1 -> Data Type Conversion5/1
  enYaw/1 -> Data Type Conversion7/1
  EnYawrate/1 -> Data Type Conversion8/1
  enForce/1 -> Data Type Conversion6/1
  "MAV_FRAME_LOCAL_NED "/1 -> Data Type Conversion9/1
  enPos/1 -> Data Type Conversion3/1
  Data Type Conversion9/1 -> Index Vector/2
  Mux5/1 -> Mux4/1
  Data Type Conversion10/1 -> Index Vector/3
  Data Type Conversion15/1 -> Mux1/4  "coordinate_frame"
  Constant/1 -> Mux2/3  "uint8 (char) Payload[80:111]"
  Data Type Conversion18/1 -> Package Head/1
  Clock/1 -> Gain/1
  len/1 -> Data Type Conversion19/1
  Data Type Conversion17/1 -> Byte Pack/2
  Data Type Conversion14/1 -> Mux1/3  "type_mask"
  Mux1/1 -> Byte Pack/1
  Package Head/1 -> Mux2/1  "int (int32) TargetType & len"
  Mux4/1 -> Data Type Conversion17/1
  TargetType/1 -> Data Type Conversion18/1
  Mux2/1 -> CmdUDP/1
  CopterID/1 -> Data Type Conversion1/1
  Gain/1 -> Data Type Conversion2/1  "timestamp"
  Data Type Conversion19/1 -> Package Head/2
  pos/1 -> Mux5/1
  Byte Pack/1 -> Mux2/2  "uint8 (char) Payload[0:79]"
  Data Type Conversion13/1 -> Index Vector/6
  Data Type Conversion12/1 -> Index Vector/5
  reserveCtrl/1 -> Mux4/2
  acc/1 -> Mux5/3
  FrameIndex/1 -> Index Vector/1
  Index Vector/1 -> Data Type Conversion15/1
  MAV_FRAME_LOCAL_NED/1 -> Data Type Conversion13/1
  MAV_FRAME_LOCAL_OFFSET_NED/1 -> Data Type Conversion10/1
  Data Type Conversion11/1 -> Index Vector/4
  "MAV_FRAME_BODY_OFFSET_NED "/1 -> Data Type Conversion12/1
  enVel/1 -> Data Type Conversion4/1
  yaw/1 -> Mux5/4
  yawrate/1 -> Mux5/5
  Data Type Conversion1/1 -> Mux1/2
  Data Type Conversion2/1 -> Mux1/1

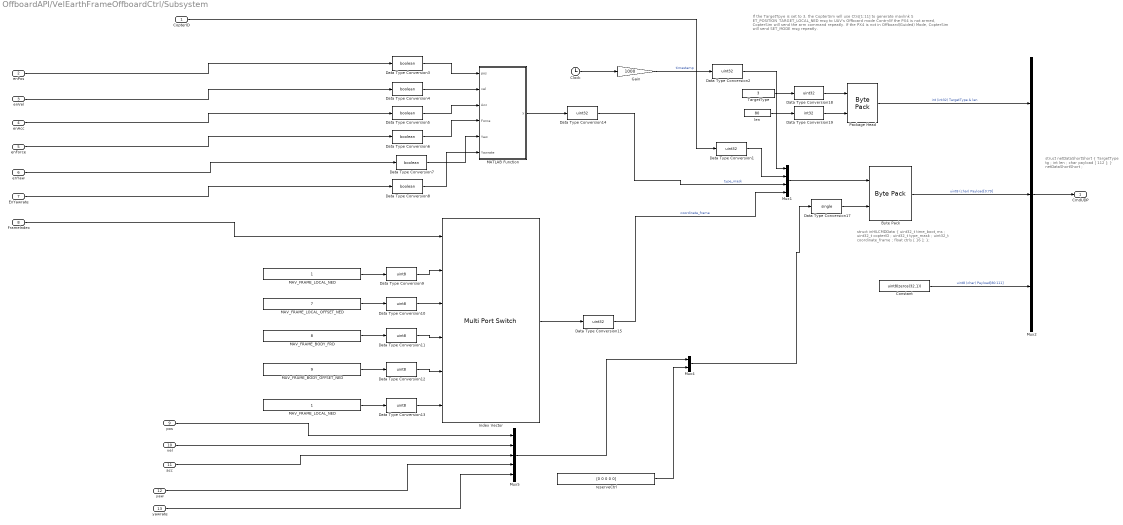
== system OffboardAPI/VelEarthFrameOffboardCtrl/Subsystem ==
  note: struct netDataShortShort {
      | TargetType tg ;
      | int len ;
      | char payload [ 112 ];
      | } netDataShortShort ;
  note: struct inHILCMDData {
      | uint32_t time_boot_ms ;
      | uint32_t copterID ;
      | uint32_t type_mask ;
      | uint32_t coordinate_frame ;
      | float ctrls [ 16 ];
      | };
  note: If the TargetTpye is set to 3, the CopterSim will use Ctrs[1:11] to generate mavlink S ET_POSITION_TARGET_LOCAL_NED msg to UAV's Offboard mode Control，
      | If the PX4 is not armed, CopterSim will send the arm command repeatly. If the PX4 is not in Offboard(Guided) Mode, CopterSim will send SET_MODE msg repeatly.
  CopterID : Inport
  enPos : Inport  Port=2
  enVel : Inport  Port=3
  enAcc : Inport  Port=4
  enForce : Inport  Port=5
  enYaw : Inport  Port=6
  EnYawrate : Inport  Port=7
  FrameIndex : Inport  Port=8
  pos : Inport  Port=9  PortDimensions=3
  vel : Inport  Port=10  PortDimensions=3
  acc : Inport  Port=11  PortDimensions=3
  yaw : Inport  Port=12  PortDimensions=1
  yawrate : Inport  Port=13  PortDimensions=1
  Byte Pack : etargetslib/Byte Pack  datatypes={'uint32','single'}  byteAlign=1
  Clock : Clock
  Constant : Constant  Value=uint8(zeros(32,1))
  Data Type Conversion{1,14..15,18} (4 alike) : DataTypeConversion  OutDataTypeStr=uint32
  Data Type Conversion{9..13} (5 alike) : DataTypeConversion  OutDataTypeStr=uint8
  Data Type Conversion17 : DataTypeConversion  OutDataTypeStr=single  LockScale=on
  Data Type Conversion19 : DataTypeConversion  OutDataTypeStr=int32
  Data Type Conversion2 : DataTypeConversion  OutDataTypeStr=uint32  RndMeth=Round
  Data Type Conversion{3..8} (6 alike) : DataTypeConversion  OutDataTypeStr=boolean
  Gain : Gain  Gain=1000
  Index Vector : MultiPortSwitch  DataPortOrder=Zero-based contiguous  Inputs=5  zeroidx=on
  MATLAB Function : MATLAB Function  TreatAsAtomicUnit=on
  MAV_FRAME_BODY_FRD : Constant  Value=8
  "MAV_FRAME_BODY_OFFSET_NED " : Constant  Value=9
  MAV_FRAME_LOCAL_NED : Constant
  "MAV_FRAME_LOCAL_NED " : Constant
  MAV_FRAME_LOCAL_OFFSET_NED : Constant  Value=7
  Mux1 : Mux
  Mux2 : Mux  Inputs=3
  Mux4 : Mux  Inputs=2
  Mux5 : Mux  Inputs=5
  Package Head : etargetslib/Byte Pack  datatypes={'uint32','int32'}  byteAlign=4
  TargetType : Constant  Value=3  OutDataTypeStr=Inherit: Inherit via back propagation
  len : Constant  Value=80  OutDataTypeStr=Inherit: Inherit via back propagation
  reserveCtrl : Constant  Value=[0 0 0 0 0]
  CmdUDP : Outport  VectorParamsAs1DForOutWhenUnconnected=off
  wires:
  Data Type Conversion7/1 -> MATLAB Function/5(Yaw)
  Data Type Conversion6/1 -> MATLAB Function/4(Force)
  MATLAB Function/1(y) -> Data Type Conversion14/1
  vel/1 -> Mux5/2
  MAV_FRAME_BODY_FRD/1 -> Data Type Conversion11/1
  Data Type Conversion3/1 -> MATLAB Function/1(pos)
  Data Type Conversion5/1 -> MATLAB Function/3(Acc)
  Data Type Conversion4/1 -> MATLAB Function/2(vel)
  Data Type Conversion8/1 -> MATLAB Function/6(Yawrate)
  enAcc/1 -> Data Type Conversion5/1
  enYaw/1 -> Data Type Conversion7/1
  EnYawrate/1 -> Data Type Conversion8/1
  enForce/1 -> Data Type Conversion6/1
  "MAV_FRAME_LOCAL_NED "/1 -> Data Type Conversion9/1
  enPos/1 -> Data Type Conversion3/1
  Data Type Conversion9/1 -> Index Vector/2
  Mux5/1 -> Mux4/1
  Data Type Conversion10/1 -> Index Vector/3
  Data Type Conversion15/1 -> Mux1/4  "coordinate_frame"
  Constant/1 -> Mux2/3  "uint8 (char) Payload[80:111]"
  Data Type Conversion18/1 -> Package Head/1
  Clock/1 -> Gain/1
  len/1 -> Data Type Conversion19/1
  Data Type Conversion17/1 -> Byte Pack/2
  Data Type Conversion14/1 -> Mux1/3  "type_mask"
  Mux1/1 -> Byte Pack/1
  Package Head/1 -> Mux2/1  "int (int32) TargetType & len"
  Mux4/1 -> Data Type Conversion17/1
  TargetType/1 -> Data Type Conversion18/1
  Mux2/1 -> CmdUDP/1
  CopterID/1 -> Data Type Conversion1/1
  Gain/1 -> Data Type Conversion2/1  "timestamp"
  Data Type Conversion19/1 -> Package Head/2
  pos/1 -> Mux5/1
  Byte Pack/1 -> Mux2/2  "uint8 (char) Payload[0:79]"
  Data Type Conversion13/1 -> Index Vector/6
  Data Type Conversion12/1 -> Index Vector/5
  reserveCtrl/1 -> Mux4/2
  acc/1 -> Mux5/3
  FrameIndex/1 -> Index Vector/1
  Index Vector/1 -> Data Type Conversion15/1
  MAV_FRAME_LOCAL_NED/1 -> Data Type Conversion13/1
  MAV_FRAME_LOCAL_OFFSET_NED/1 -> Data Type Conversion10/1
  Data Type Conversion11/1 -> Index Vector/4
  "MAV_FRAME_BODY_OFFSET_NED "/1 -> Data Type Conversion12/1
  enVel/1 -> Data Type Conversion4/1
  yaw/1 -> Mux5/4
  yawrate/1 -> Mux5/5
  Data Type Conversion1/1 -> Mux1/2
  Data Type Conversion2/1 -> Mux1/1

== matlab function OffboardAPI/VelEarthFrameOffboardCtrl/Subsystem/MATLAB Function ==
  data: pos input; y output; vel input; Acc input; Force input; Yaw input; Yawrate input
function y = fcn(pos,vel,Acc,Force,Yaw,Yawrate)
y=uint32(0);
if ~pos
    y = bitor(y,uint32(7));
end

if~vel
    y = bitor(y,bitshift(uint32(7),3));
end

if ~Acc
    y = bitor(y,bitshift(uint32(7),6));
end

if Force
    y = bitor(y,bitshift(uint32(1),9));
end

if ~Yaw
    y = bitor(y,bitshift(uint32(1),10));
end

if ~Yawrate
    y = bitor(y,bitshift(uint32(1),11));
end

== matlab function OffboardAPI/UDP_SIL_State_Receiver/DataValidation ==
  data: inGPSPos input; outGPSPos output; inGpsVel input; inEulerAng input; outGpsVel output; outEulerAng output; outDataOk output
function [outGPSPos,outGpsVel,outEulerAng,outDataOk] = fcn(inGPSPos,inGpsVel,inEulerAng)

outGPSPos = [0;0;0];
outGpsVel = [0;0;0];
outEulerAng = [0;0;0];
outDataOk = 0;

if(abs(inGPSPos(1))<10000)
    outGPSPos=inGPSPos;
    outGpsVel=inGpsVel;
    outEulerAng = inEulerAng;
    outDataOk = 1;
end

== matlab function OffboardAPI/VelBodyFrameOffboardCtrl/Subsystem/MATLAB Function ==
  data: pos input; y output; vel input; Acc input; Force input; Yaw input; Yawrate input
function y = fcn(pos,vel,Acc,Force,Yaw,Yawrate)
y=uint32(0);
if ~pos
    y = bitor(y,uint32(7));
end

if~vel
    y = bitor(y,bitshift(uint32(7),3));
end

if ~Acc
    y = bitor(y,bitshift(uint32(7),6));
end

if Force
    y = bitor(y,bitshift(uint32(1),9));
end

if ~Yaw
    y = bitor(y,bitshift(uint32(1),10));
end

if ~Yawrate
    y = bitor(y,bitshift(uint32(1),11));
end

== matlab function OffboardAPI/PosTargetEarthFrameOffboardCtrl/Subsystem/MATLAB Function ==
  data: pos input; y output; vel input; Acc input; Force input; Yaw input; Yawrate input
function y = fcn(pos,vel,Acc,Force,Yaw,Yawrate)
y=uint32(0);
if ~pos
    y = bitor(y,uint32(7));
end

if~vel
    y = bitor(y,bitshift(uint32(7),3));
end

if ~Acc
    y = bitor(y,bitshift(uint32(7),6));
end

if Force
    y = bitor(y,bitshift(uint32(1),9));
end

if ~Yaw
    y = bitor(y,bitshift(uint32(1),10));
end

if ~Yawrate
    y = bitor(y,bitshift(uint32(1),11));
end

== matlab function OffboardAPI/UDP_True_State_Receiver/VehicleDataPerse ==
  data: Data input; y output uint8 size=[152,1]; Length input; dataOk output
function [y,dataOk] = fcn(Data,Length)
y=uint8(zeros(152,1));
dataOk = 0;
if Length ~= 200
    return;
end
len = typecast(Data(5:8), 'int32');

if len ~= 152
   return; 
end

y = Data(9:160);
dataOk = 1;

== matlab function OffboardAPI/UDP_SIL_State_Receiver/VehicleDataPerse ==
  data: Data input; y output uint8; Length input; dataOk output
function [y,dataOk] = fcn(Data,Length)
y=uint8(zeros(112,1));
dataOk = 0;
if Length ~= 120
    return;
end
len = typecast(Data(5:8), 'int32');

if len ~= 112
   return; 
end

y = Data(9:120);
dataOk = 1;
